simulink model "LSProj2015"  (R2022a)
settings: Solver=VariableStepAuto  StartTime=0.0  StopTime=10  RelTol=1e-3
settings Model: Creator=sanam  LastModifiedBy=sanam
settings SolverCC: AlgebraicLoopSolver=TrustRegion
settings OptimizationCC: LifeSpan=inf
settings DebuggingCC: SFExecutionAtInitializationDiag=none  SFMachineParentedDataDiag=warning  ArithmeticOperatorsInVariantConditions=warning
settings SFSimCC: CustomCodeUndefinedFunction=UseInterfaceOnly
settings CodeAppCC: StateflowObjectComments=on

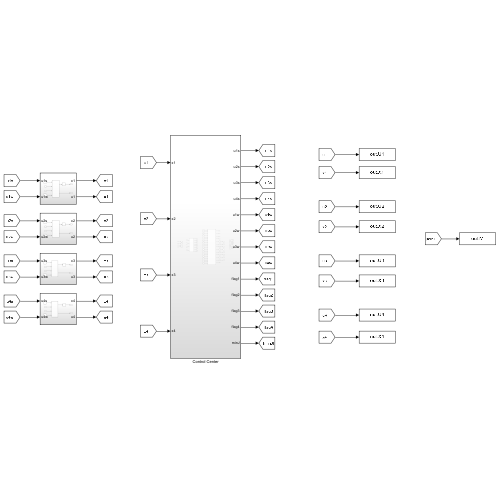
[thumbnail: Simulink's stored preview of the top-level diagram]
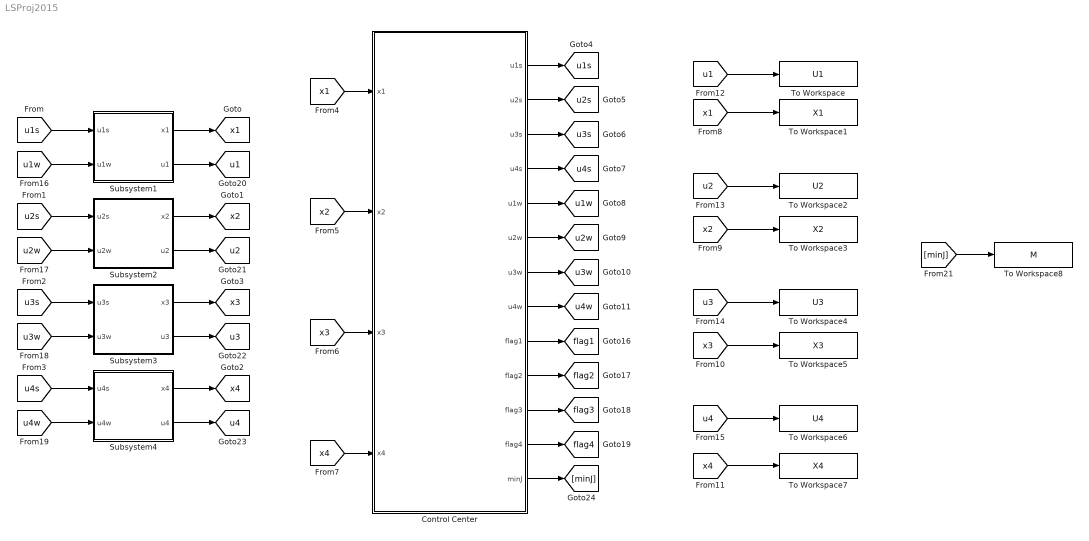
== system LSProj2015 ==
  Control Center : Subsystem
  Subsystem1 : Subsystem
  Subsystem2 : Subsystem
  Subsystem3 : Subsystem
  Subsystem4 : Subsystem
  To Workspace : ToWorkspace  VariableName=U1  SaveFormat=Timeseries  SampleTime=-1
  To Workspace1 : ToWorkspace  VariableName=X1  SaveFormat=Timeseries  SampleTime=-1
  To Workspace2 : ToWorkspace  VariableName=U2  SaveFormat=Timeseries  SampleTime=-1
  To Workspace3 : ToWorkspace  VariableName=X2  SaveFormat=Timeseries  SampleTime=-1
  To Workspace4 : ToWorkspace  VariableName=U3  SaveFormat=Timeseries  SampleTime=-1
  To Workspace5 : ToWorkspace  VariableName=X3  SaveFormat=Timeseries  SampleTime=-1
  To Workspace6 : ToWorkspace  VariableName=U4  SaveFormat=Timeseries  SampleTime=-1
  To Workspace7 : ToWorkspace  VariableName=X4  SaveFormat=Timeseries  SampleTime=-1
  To Workspace8 : ToWorkspace  VariableName=M  SaveFormat=Timeseries  SampleTime=-1
  tag scope: flag1=global, flag2=global, flag3=global, flag4=global, u1=global, u1s=global, u1w=global, u2=global, u2s=global, u2w=global, u3=global, u3s=global, u3w=global, u4=global, u4s=global, u4w=global, x1=global, x2=global, x3=global, x4=global
  wires:
  Subsystem1/1(x1) -> [x1]
  Control Center/1(u1s) -> [u1s]
  Control Center/2(u2s) -> [u2s]
  Control Center/3(u3s) -> [u3s]
  Control Center/4(u4s) -> [u4s]
  [u1s] -> Subsystem1/1(u1s)
  Control Center/8(u4w) -> [u4w]
  Control Center/5(u1w) -> [u1w]
  Control Center/7(u3w) -> [u3w]
  Control Center/6(u2w) -> [u2w]
  [u1w] -> Subsystem1/2(u1w)
  Control Center/10(flag2) -> [flag2]
  Control Center/9(flag1) -> [flag1]
  Control Center/11(flag3) -> [flag3]
  Control Center/12(flag4) -> [flag4]
  [u3s] -> Subsystem3/1(u3s)
  [u3w] -> Subsystem3/2(u3w)
  Subsystem3/1(x3) -> [x3]
  Subsystem4/1(x4) -> [x4]
  [u4s] -> Subsystem4/1(u4s)
  [u4w] -> Subsystem4/2(u4w)
  [x4] -> Control Center/4(x4)
  [x3] -> Control Center/3(x3)
  [x2] -> Control Center/2(x2)
  [x1] -> Control Center/1(x1)
  [u2s] -> Subsystem2/1(u2s)
  [u2w] -> Subsystem2/2(u2w)
  Subsystem2/1(x2) -> [x2]
  [x1] -> To Workspace1/1
  [x2] -> To Workspace3/1
  [u1] -> To Workspace/1
  Subsystem1/2(u1) -> [u1]
  Subsystem2/2(u2) -> [u2]
  Subsystem3/2(u3) -> [u3]
  Subsystem4/2(u4) -> [u4]
  [u2] -> To Workspace2/1
  Control Center/13(minJ) -> [minJ]
  [u3] -> To Workspace4/1
  [x3] -> To Workspace5/1
  [x4] -> To Workspace7/1
  [u4] -> To Workspace6/1
  [minJ] -> To Workspace8/1

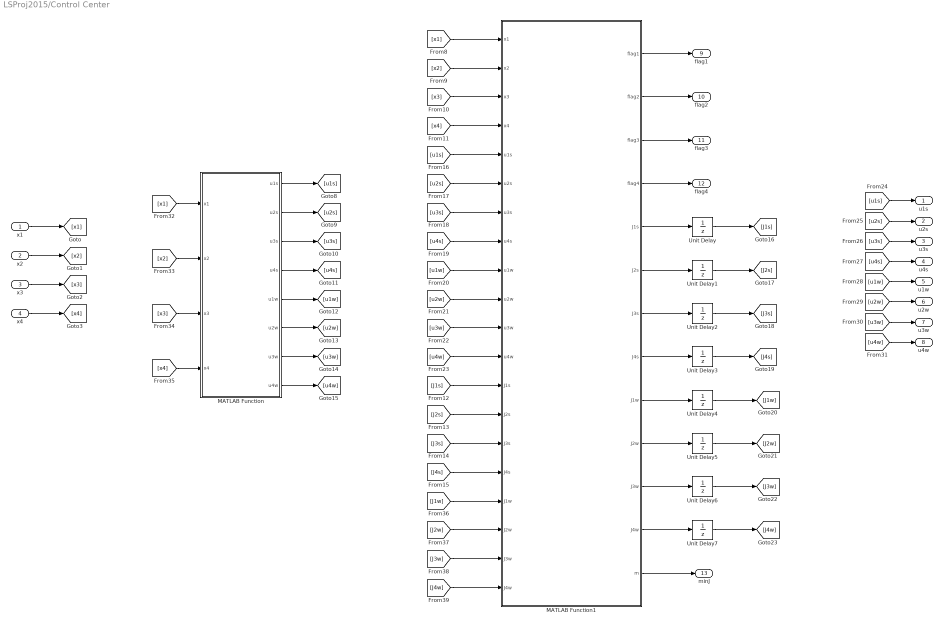
== system LSProj2015/Control Center ==
  x1 : Inport
  x2 : Inport  Port=2
  x3 : Inport  Port=3
  x4 : Inport  Port=4
  MATLAB Function : MATLAB Function  TreatAsAtomicUnit=on
  MATLAB Function1 : MATLAB Function  TreatAsAtomicUnit=on
  Unit Delay{,1..7} (8 alike) : UnitDelay  SampleTime=-1  HasFrameUpgradeWarning=on
  u1s : Outport
  u2s : Outport  Port=2
  u3s : Outport  Port=3
  u4s : Outport  Port=4
  u1w : Outport  Port=5
  u2w : Outport  Port=6
  u3w : Outport  Port=7
  u4w : Outport  Port=8
  flag1 : Outport  Port=9
  flag2 : Outport  Port=10
  flag3 : Outport  Port=11
  flag4 : Outport  Port=12
  minJ : Outport  Port=13
  wires:
  x1/1 -> [x1]
  x2/1 -> [x2]
  x3/1 -> [x3]
  x4/1 -> [x4]
  MATLAB Function/1(u1s) -> [u1s]
  MATLAB Function/2(u2s) -> [u2s]
  MATLAB Function/3(u3s) -> [u3s]
  MATLAB Function/4(u4s) -> [u4s]
  MATLAB Function/5(u1w) -> [u1w]
  MATLAB Function/6(u2w) -> [u2w]
  MATLAB Function/7(u3w) -> [u3w]
  MATLAB Function/8(u4w) -> [u4w]
  [u1s] -> u1s/1
  [u2w] -> u2w/1
  [u3s] -> u3s/1
  [u1w] -> u1w/1
  [u2s] -> u2s/1
  [u4s] -> u4s/1
  [u3w] -> u3w/1
  [u4w] -> u4w/1
  MATLAB Function1/1(flag1) -> flag1/1
  MATLAB Function1/2(flag2) -> flag2/1
  MATLAB Function1/3(flag3) -> flag3/1
  MATLAB Function1/4(flag4) -> flag4/1
  [x1] -> MATLAB Function/1(x1)
  [x2] -> MATLAB Function/2(x2)
  [x3] -> MATLAB Function/3(x3)
  [x4] -> MATLAB Function/4(x4)
  [u4w] -> MATLAB Function1/12(u4w)
  [u3w] -> MATLAB Function1/11(u3w)
  [u2w] -> MATLAB Function1/10(u2w)
  [u1w] -> MATLAB Function1/9(u1w)
  [u4s] -> MATLAB Function1/8(u4s)
  [u3s] -> MATLAB Function1/7(u3s)
  [u2s] -> MATLAB Function1/6(u2s)
  [u1s] -> MATLAB Function1/5(u1s)
  [x4] -> MATLAB Function1/4(x4)
  [x3] -> MATLAB Function1/3(x3)
  [x2] -> MATLAB Function1/2(x2)
  [x1] -> MATLAB Function1/1(x1)
  MATLAB Function1/5(J1s) -> Unit Delay/1
  MATLAB Function1/6(J2s) -> Unit Delay1/1
  MATLAB Function1/7(J3s) -> Unit Delay2/1
  MATLAB Function1/8(J4s) -> Unit Delay3/1
  MATLAB Function1/9(J1w) -> Unit Delay4/1
  MATLAB Function1/10(J2w) -> Unit Delay5/1
  MATLAB Function1/11(J3w) -> Unit Delay6/1
  MATLAB Function1/12(J4w) -> Unit Delay7/1
  [J1s] -> MATLAB Function1/13("J1s ")
  [J2s] -> MATLAB Function1/14("J2s ")
  [J3s] -> MATLAB Function1/15("J3s ")
  [J4s] -> MATLAB Function1/16("J4s ")
  [J1w] -> MATLAB Function1/17("J1w ")
  [J2w] -> MATLAB Function1/18("J2w ")
  [J3w] -> MATLAB Function1/19("J3w ")
  [J4w] -> MATLAB Function1/20("J4w ")
  Unit Delay/1 -> [J1s]
  Unit Delay1/1 -> [J2s]
  Unit Delay7/1 -> [J4w]
  Unit Delay6/1 -> [J3w]
  Unit Delay5/1 -> [J2w]
  Unit Delay4/1 -> [J1w]
  Unit Delay3/1 -> [J4s]
  Unit Delay2/1 -> [J3s]
  MATLAB Function1/13(m) -> minJ/1

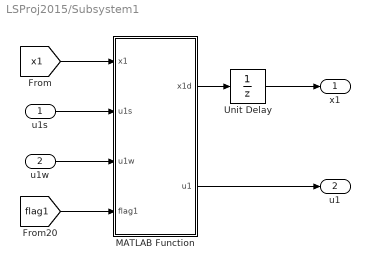
== system LSProj2015/Subsystem1 ==
  u1s : Inport
  u1w : Inport  Port=2
  MATLAB Function : MATLAB Function  TreatAsAtomicUnit=on
  Unit Delay : UnitDelay  InitialCondition=[1.5;1.5]  HasFrameUpgradeWarning=on
  x1 : Outport
  u1 : Outport  Port=2
  wires:
  MATLAB Function/1(x1d) -> Unit Delay/1
  Unit Delay/1 -> x1/1
  [x1] -> MATLAB Function/1(x1)
  u1s/1 -> MATLAB Function/2(u1s)
  u1w/1 -> MATLAB Function/3(u1w)
  [flag1] -> MATLAB Function/4(flag1)
  MATLAB Function/2(u1) -> u1/1

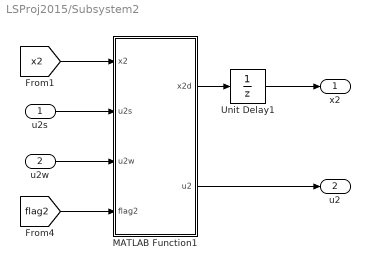
== system LSProj2015/Subsystem2 ==
  u2s : Inport
  u2w : Inport  Port=2
  MATLAB Function1 : MATLAB Function  TreatAsAtomicUnit=on
  Unit Delay1 : UnitDelay  InitialCondition=[1.5;1.5]  HasFrameUpgradeWarning=on
  x2 : Outport
  u2 : Outport  Port=2
  wires:
  Unit Delay1/1 -> x2/1
  [x2] -> MATLAB Function1/1(x2)
  [flag2] -> MATLAB Function1/4(flag2)
  u2s/1 -> MATLAB Function1/2(u2s)
  u2w/1 -> MATLAB Function1/3(u2w)
  MATLAB Function1/1(x2d) -> Unit Delay1/1
  MATLAB Function1/2(u2) -> u2/1

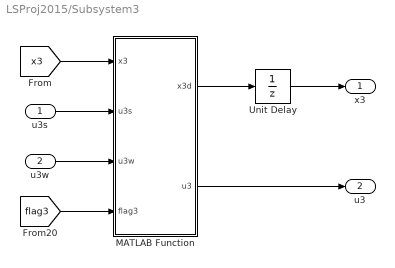
== system LSProj2015/Subsystem3 ==
  u3s : Inport
  u3w : Inport  Port=2
  MATLAB Function : MATLAB Function  TreatAsAtomicUnit=on
  Unit Delay : UnitDelay  InitialCondition=[1.5;1.5]  HasFrameUpgradeWarning=on
  x3 : Outport
  u3 : Outport  Port=2
  wires:
  MATLAB Function/1(x3d) -> Unit Delay/1
  [x3] -> MATLAB Function/1(x3)
  u3s/1 -> MATLAB Function/2(u3s)
  u3w/1 -> MATLAB Function/3(u3w)
  [flag3] -> MATLAB Function/4(flag3)
  Unit Delay/1 -> x3/1
  MATLAB Function/2(u3) -> u3/1

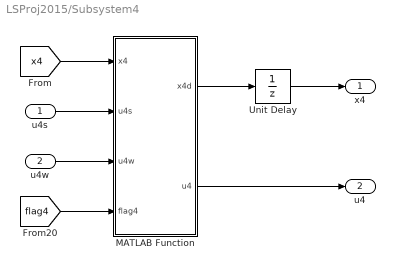
== system LSProj2015/Subsystem4 ==
  u4s : Inport
  u4w : Inport  Port=2
  MATLAB Function : MATLAB Function  TreatAsAtomicUnit=on
  Unit Delay : UnitDelay  InitialCondition=[1.5;1.5]  HasFrameUpgradeWarning=on
  x4 : Outport
  u4 : Outport  Port=2
  wires:
  Unit Delay/1 -> x4/1
  u4w/1 -> MATLAB Function/3(u4w)
  MATLAB Function/1(x4d) -> Unit Delay/1
  [x4] -> MATLAB Function/1(x4)
  [flag4] -> MATLAB Function/4(flag4)
  u4s/1 -> MATLAB Function/2(u4s)
  MATLAB Function/2(u4) -> u4/1

== matlab function LSProj2015/Control Center/MATLAB Function ==
  data: x1 input; u1s output; x2 input; x3 input; x4 input; u2s output; u3s output; u4s output; u1w output; u2w output; u3w output; u4w output
function [u1s,u2s,u3s,u4s,u1w,u2w,u3w,u4w] = fcn(x1,x2,x3,x4)

coder.extrinsic("dlqr")



A1=[-3 -2; 1 0];
B1=[4; 0];


A2=[-5.5 -3; 2 0];
B2=[2; 0];


A3=[-4 -1.75; 1 0];
B3=[1; 0];

A4=[-4 -2; 2 0];
B4=[2; 0];

Q1=eye(2);
R1=1;


Q2=[1 0;0 2];
R2=0.5;

Q3=[2 0;0 1];
R3=1;

Q4=2*eye(2);
R4=2;

k1=zeros(1,2);
k2=zeros(1,2);
k3=zeros(1,2);
k4=zeros(1,2);

k1w=zeros(1,2);
k2w=zeros(1,2);
k3w=zeros(1,2);
k4w=zeros(1,2);

k1=dlqr(A1,B1,Q1,R1);

k2=dlqr(A2,B2,Q2,R2);

k3=dlqr(A3,B3,Q3,R3);

k4=dlqr(A4,B4,Q4,R4);


k1w=dlqr(A1,B1,Q4,R4);

k2w=dlqr(A2,B2,Q1,R1);

k3w=dlqr(A3,B3,Q2,R2);

k4w=dlqr(A4,B4,Q3,R3);


u1s=-k1*x1;

u2s=-k2*x2;

u3s=-k3*x3;

u4s=-k4*x4;


u1w=-k1w*x1;

u2w=-k2w*x2;

u3w=-k3w*x3;

u4w=-k4w*x4;


end

== matlab function LSProj2015/Subsystem3/MATLAB Function ==
  data: x3 input; x3d output; u3s input; u3w input; flag3 input; u3 output
function [x3d,u3]  = fcn(x3,u3s,u3w,flag3)


if flag3==1
    u3=u3s;
else
    u3=u3w;
end

A3=[-4 -1.75; 1 0];
B3=[1; 0];


x3d= A3*x3 + B3*u3;


end

== matlab function LSProj2015/Subsystem2/MATLAB Function1 ==
  data: x2 input; x2d output; u2s input; u2w input; flag2 input; u2 output
function [x2d,u2] = fcn(x2,u2s,u2w,flag2)


if flag2==1
    u2=u2s;
else
    u2=u2w;
end



A2=[-5.5 -3; 2 0];
B2=[2; 0];

x2d= A2*x2 + B2*u2;


end

== matlab function LSProj2015/Subsystem4/MATLAB Function ==
  data: x4 input; x4d output; u4s input; u4w input; flag4 input; u4 output
function [x4d,u4]  = fcn(x4,u4s,u4w,flag4)


if flag4==1
    u4=u4s;
else
    u4=u4w;
end


A4=[-4 -2; 2 0];
B4=[2; 0];


x4d= A4*x4 + B4*u4;


end

== matlab function LSProj2015/Subsystem1/MATLAB Function ==
  data: x1 input; x1d output; u1s input; u1w input; flag1 input; u1 output
function [x1d,u1] = fcn(x1,u1s,u1w,flag1)


if flag1==1
    u1=u1s;
else
    u1=u1w;
end


A1=[-3 -2; 1 0];
B1=[4; 0];


x1d= A1*x1 + B1*u1;


end

== matlab function LSProj2015/Control Center/MATLAB Function1 ==
  data: x1 input; x2 input; x3 input; x4 input; u1s input; u2s input; u3s input; u4s input; u1w input; u2w input; u3w input; u4w input; flag1 output; flag2 output; flag3 output; flag4 output; J1s input; J2s input; J3s input; J4s input; J1w input; J2w input; J3w input; J4w input; J1s output; J2s output; J3s output; J4s output; J1w output; J2w output; J3w output; J4w output; m output
function [flag1,flag2,flag3,flag4,J1s,J2s,J3s,J4s,J1w,J2w,J3w,J4w,m]= fcn(x1,x2,x3,x4,u1s,u2s,u3s,u4s,u1w,u2w,u3w,u4w,J1s,J2s,J3s,J4s,J1w,J2w,J3w,J4w)

coder.extrinsic("allcomb")


Q1=eye(2);
R1=1;

Q2=[1 0;0 2];
R2=0.5;

Q3=[2 0;0 1];
R3=1;

Q4=2*eye(2);
R4=2;


J1s= J1s+  x1'*Q1*x1 + u1s'*R1*u1s;
J2s= J2s+ x2'*Q2*x2 + u2s'*R2*u2s;
J3s= J3s+ x3'*Q3*x3 + u3s'*R3*u3s;
J4s= J4s+ x4'*Q4*x4 + u4s'*R4*u4s;

J1w= J1w+ x1'*Q1*x1 + u1w'*R1*u1w;
J2w= J2w+ x2'*Q2*x2 + u2w'*R2*u2w;
J3w= J3w+ x3'*Q3*x3 + u3w'*R3*u3w;
J4w= J4w+ x4'*Q4*x4 + u4w'*R4*u4w;

comb=zeros(16,4);

comb=allcomb([J1s J1w],[J2s J2w],[J3s J3w],[J4s J4w]);


s=sum(comb,2);

[m,i]=min(s);

mincomb=comb(i,:);


dec1=mincomb(1);
dec2=mincomb(2);
dec3=mincomb(3);
dec4=mincomb(4);


if dec1==J1s
    flag1=1;
else
    flag1=2;
end
  


if dec2==J2s
    flag2=1;
else
    flag2=2;
end



if dec3==J3s
    flag3=1;
else
    flag3=2;
end



if dec4==J4s
    flag4=1;
else
    flag4=2;
end




end
